simulink model "castro2020"  (R2025b)
settings: Solver=ode15s  StopTime=10  MaxStep=1e-3
libraries: slpidlib x1, simulink x1
settings DataIOCC: SaveOutput=off  SignalLogging=off  DSMLogging=off  ReturnWorkspaceOutputs=off  TimeSaveName=t
settings DebuggingCC: AlgebraicLoopMsg=none  ArtificialAlgebraicLoopMsg=none  MaxConsecutiveZCsMsg=none  OperatingPointInterfaceChecksumMismatchMsg=none

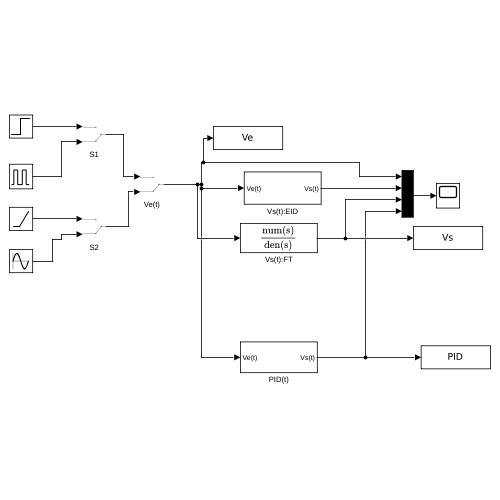
[thumbnail: Simulink's stored preview of the top-level diagram]
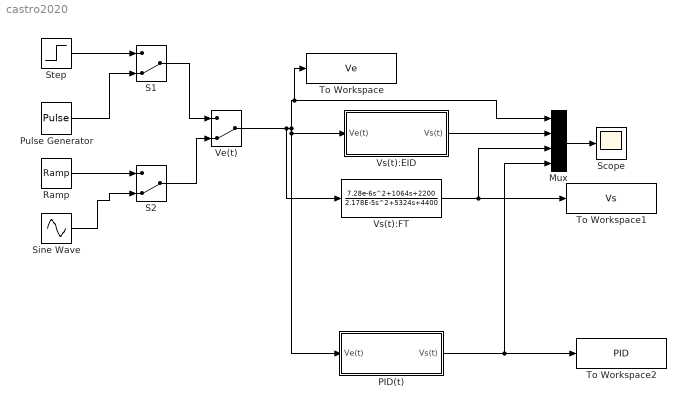
== system castro2020 ==
  Mux : Mux
  PID(t) : Subsystem
  Pulse Generator : DiscretePulseGenerator  PulseType=Time based  Period=10  PulseWidth=10  PhaseDelay=1
  Ramp : simulink/Sources/Ramp  slope=1/10  start=0  InitialOutput=0
  S1 : ManualSwitch  CurrentSetting=0
  S2 : ManualSwitch  CurrentSetting=0
  Scope : Scope
      settings: ActiveDisplayYMinimum=-1.1929119540864606  ActiveDisplayYMaximum=1.4589275731821982
  Sine Wave : Sin  Frequency=pi/2  SampleTime=0
  Step : Step  Time=0  Before=1  SampleTime=0
  To Workspace : ToWorkspace  VariableName=Ve  SampleTime=-1
  To Workspace1 : ToWorkspace  VariableName=Vs  SampleTime=-1
  To Workspace2 : ToWorkspace  VariableName=PID  SampleTime=-1
  Ve(t) : ManualSwitch  CurrentSetting=0
  Vs(t):EID : Subsystem
  Vs(t):FT : TransferFcn  Numerator=[7.28e-6,1064,2200]  Denominator=[2.178E-5,5324,4400]
  wires:
  Mux/1 -> Scope/1
  Step/1 -> S1/1
  Pulse Generator/1 -> S1/2
  Ramp/1 -> S2/1
  Sine Wave/1 -> S2/2
  S1/1 -> Ve(t)/1
  S2/1 -> Ve(t)/2
  Ve(t)/1 -> PID(t)/1(Ve(t)), Vs(t):EID/1(Ve(t)), To Workspace/1, Mux/1, Vs(t):FT/1
  Vs(t):EID/1(Vs(t)) -> Mux/2
  Vs(t):FT/1 -> To Workspace1/1, Mux/3
  PID(t)/1(Vs(t)) -> To Workspace2/1, Mux/4

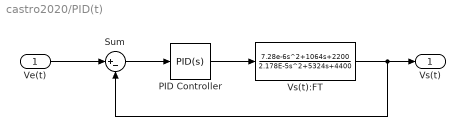
== system castro2020/PID(t) ==
  Ve(t) : Inport
  PID Controller : slpidlib/PID Controller  Controller=PID  Form=Parallel  TimeDomain=Continuous-time  UseExternalTs=off  SampleTime=-1  IntegratorMethod=Forward Euler  FilterMethod=Forward Euler  ControllerParametersSource=internal  P=12.7636  I=851.3046  UseKiTs=off  D=-0.4532  UseExternalDerivativeSource=off  N=28.1634  UseFilter=on  TunerSelectOption=Transfer Function Based (PID Tuner App)  InitialConditionSource=internal  InitialConditionForIntegrator=0  InitialConditionForFilter=0  DifferentiatorICPrevScaledInput=0  ExternalReset=none  TrackingMode=off  Kt=1  LimitOutput=off  SatLimitsSource=internal  UpperSaturationLimit=inf  LowerSaturationLimit=-inf  LinearizeAsGain=on  AntiWindupMode=none  Kb=1  LimitIntegrator=off  UpperIntegratorSaturationLimit=inf  LowerIntegratorSaturationLimit=-inf  POutMin=[]  POutMax=[]  IOutMin=[]  IOutMax=[]  DOutMin=[]  DOutMax=[]  NOutMin=[]  NOutMax=[]  SumOutMin=[]  SumOutMax=[]  SaturationOutMin=[]  SaturationOutMax=[]  PParamMin=[]  PParamMax=[]  IParamMin=[]  IParamMax=[]  DParamMin=[]  DParamMax=[]  NParamMin=[]  NParamMax=[]  KbParamMin=[]  KbParamMax=[]  KtParamMin=[]  KtParamMax=[]  KbOutMin=[]  KbOutMax=[]  KtOutMin=[]  KtOutMax=[]  IntegratorOutMin=[]  IntegratorOutMax=[]  FilterOutMin=[]  FilterOutMax=[]  SumI1OutMin=[]  SumI1OutMax=[]  SumI2OutMin=[]  SumI2OutMax=[]  SumI3OutMin=[]  SumI3OutMax=[]  SumI4OutMin=[]  SumI4OutMax=[]  SumDOutMin=[]  SumDOutMax=[]  DifferentiatorOutMin=[]  DifferentiatorOutMax=[]  FilterDiffOutCoefMin=[]  FilterDiffOutCoefMax=[]  ReciprocalOutMin=[]  ReciprocalOutMax=[]  SumDenOutMin=[]  SumDenOutMax=[]  SumNumOutMin=[]  SumNumOutMax=[]  DivideOutMin=[]  DivideOutMax=[]  UdiffTsProdOutMin=[]  UdiffTsProdOutMax=[]  NTsProdOutMin=[]  NTsProdOutMax=[]  UintegralTsProdOutMin=[]  UintegralTsProdOutMax=[]  UngainTsProdOutMin=[]  UngainTsProdOutMax=[]  ClampingZeroOutDataTypeStr=Inherit: Inherit via back propagation  ClampingZeroOutMin=[]  ClampingZeroOutMax=[]  FilterDenConstantOutDataTypeStr=Inherit: Inherit via back propagation  FilterDenConstantOutMin=[]  FilterDenConstantOutMax=[]  PCopyOutDataTypeStr=Inherit: Inherit via back propagation  PCopyOutMin=[]  PCopyOutMax=[]  NCopyOutDataTypeStr=Inherit: Inherit via back propagation  NCopyOutMin=[]  NCopyOutMax=[]  IntegratorContinuousStateAttributes=''  IntegratorStateMustResolveToSignalObject=off  IntegratorRTWStateStorageClass=Auto  FilterContinuousStateAttributes=''  FilterStateMustResolveToSignalObject=off  FilterRTWStateStorageClass=Auto  ParallelPVariant=InternalParameters  IdealPVariant=Disabled  IVariant=InternalParameters  DVariant=InternalParameters  IntegratorVariant=Continuous  SatVariant=Disabled  AWVariant=Passthrough  PCopyVariant=Disabled  TRVariant=Disabled  FdbkBlocksVariant=Forward  IdealPFdbkVariant=Disabled  SatFdbkVariant=Disabled  DerivativeFilterVariant=ContFilter  NVariant=InternalParameters  NCopyVariant=Disabled  FilterICVariant=InternalICsFilter  IntegratorICVariant=InternalICs  ExternalResetVariant=Disabled  TRSumVariant=Passthrough  SumFdbkVariant=Disabled  SumVariant=Sum_PID  TsampFilterVariant=InternalTs  TsampNgainVariant=Passthrough  TsampIntegralVariant=Disabled_SignalSpec  ExternalSaturationOutDataTypeStr=Inherit: Same as second input  DerivativeSourceVariant=ErrorSignal  PreIntVariant=InternalPreInt
  Sum : Sum  Inputs=|+-
  Vs(t):FT : TransferFcn  Numerator=[7.28e-6,1064,2200]  Denominator=[2.178E-5,5324,4400]
  Vs(t) : Outport
  wires:
  Ve(t)/1 -> Sum/1
  Sum/1 -> PID Controller/1
  PID Controller/1 -> Vs(t):FT/1
  Vs(t):FT/1 -> Sum/2, Vs(t)/1

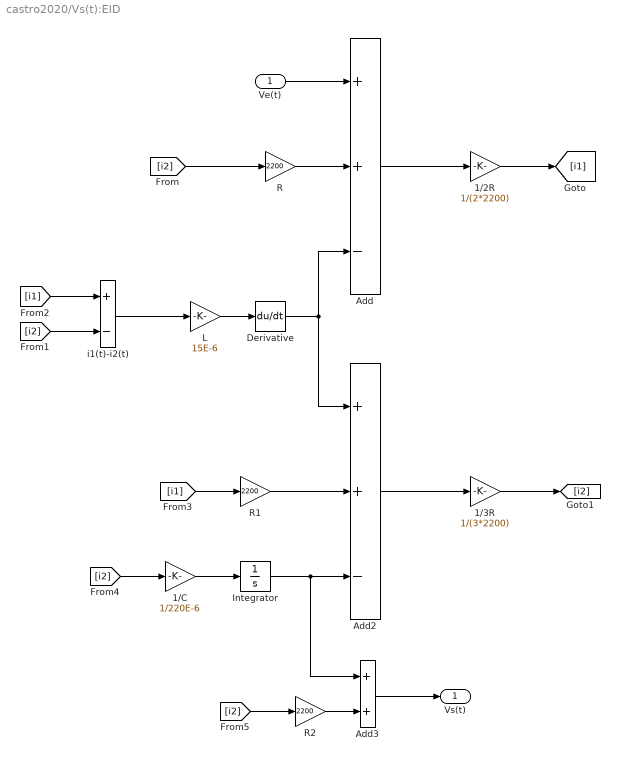
== system castro2020/Vs(t):EID ==
  Ve(t) : Inport
  1/2R : Gain  Gain=1/(2*2200)
  1/3R : Gain  Gain=1/(3*2200)
  1/C : Gain  Gain=1/220E-6
  Add : Sum  Inputs=++-
  Add2 : Sum  Inputs=++-
  Add3 : Sum
  Derivative : Derivative
  Integrator : Integrator
  L : Gain  Gain=15E-6
  R : Gain  Gain=2200
  R1 : Gain  Gain=2200
  R2 : Gain  Gain=2200
  i1(t)-i2(t) : Sum  Inputs=+-
  Vs(t) : Outport
  wires:
  Ve(t)/1 -> Add/1
  Add/1 -> 1/2R/1
  1/2R/1 -> [i1]
  [i2] -> R/1
  i1(t)-i2(t)/1 -> L/1
  L/1 -> Derivative/1
  [i2] -> i1(t)-i2(t)/2
  [i1] -> i1(t)-i2(t)/1
  Add2/1 -> 1/3R/1
  1/3R/1 -> [i2]
  Derivative/1 -> Add/3, Add2/1
  R1/1 -> Add2/2
  [i1] -> R1/1
  1/C/1 -> Integrator/1
  Integrator/1 -> Add3/1, Add2/3
  [i2] -> 1/C/1
  R2/1 -> Add3/2
  [i2] -> R2/1
  Add3/1 -> Vs(t)/1
  R/1 -> Add/2
